simulink model "Segway3"  (R2015a)
settings: Solver=ode3  SolverMode=SingleTasking  StartTime=0.0  StopTime=10.0  RelTol=1e-3
libraries: legonxtlib x12
settings Model: ExtModeTrigDuration=2  Creator=Vladimir  LastModifiedBy=Vladimir
settings OptimizationCC: OptimizeModelRefInitCode=on  LifeSpan=1
settings DebuggingCC: UnderspecifiedInitializationDetection=Classic  MergeDetectMultiDrivingBlocksExec=none
settings HardwareCC: ProdLargestAtomicInteger=Long  ProdLargestAtomicFloat=Float  ProdEndianess=LittleEndian  ProdHWDeviceType=ARM Compatible->ARM 7
settings RTWCC: SystemTargetFile=realtime.tlc  GenerateMakefile=off  TemplateMakefile=realtime.tmf  Description=Run on Target Hardware  RTWVerbose=off
settings ERTTargetCC: CombineOutputUpdateFcns=off  ExtModeTransport=2  ExtModeMexFile=ext_serial_win32_comm_no_acks_rtt  ExtModeMexArgs=0 1 9600  ERTSrcFileBannerTemplate=realtime_code_template.cgt  ERTHdrFileBannerTemplate=realtime_code_template.cgt  ERTDataSrcFileTemplate=realtime_code_template.cgt  ERTDataHdrFileTemplate=realtime_code_template.cgt  ERTCustomFileTemplate=realtime_file_process.tlc

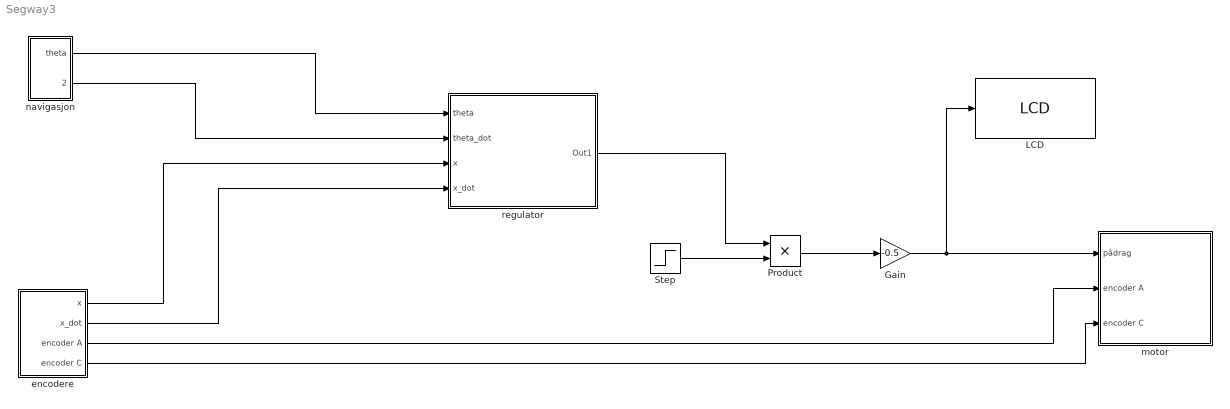
== system Segway3 ==
  Gain : Gain  Gain=-0.5
  LCD : legonxtlib/LCD  slcdStr=u  slcdLine=7  slcdFormat=Decimal  blockPlatform=LegoMindstormsNXT
  Product : Product
  Step : Step  Time=5  SampleTime=1
  encodere : Subsystem
  motor : Subsystem
  navigasjon : Subsystem
  regulator : Subsystem
  wires:
  encodere/3(encoder A) -> motor/2(encoder A)
  encodere/4("encoder C ") -> motor/3(" encoder C")
  navigasjon/1(theta) -> regulator/1(theta)
  navigasjon/2(theta_dot) -> regulator/2(theta_dot)
  encodere/1(x) -> regulator/3(x)
  encodere/2(x_dot) -> regulator/4(x_dot)
  Gain/1 -> motor/1(pådrag), LCD/1
  Step/1 -> Product/2
  regulator/1(Out1) -> Product/1
  Product/1 -> Gain/1

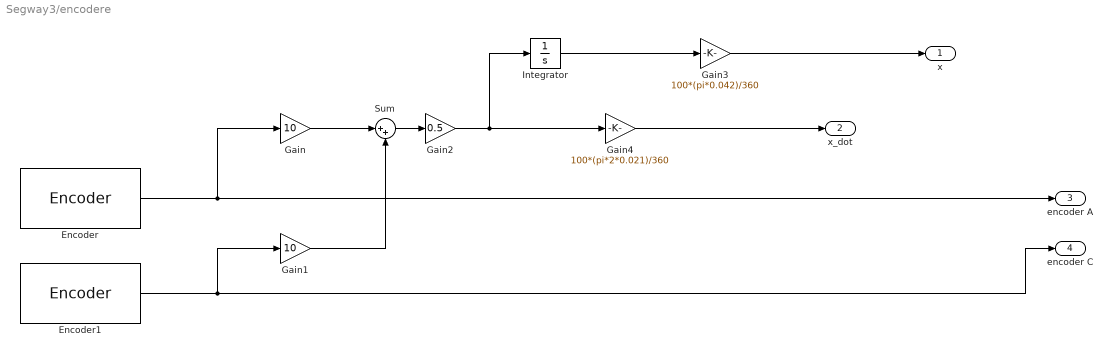
== system Segway3/encodere ==
  Encoder : legonxtlib/Encoder  portNumber=A  opMode=Reset at each sample time  sampleTime=0.1  blockPlatform=LegoMindstormsNXT
  Encoder1 : legonxtlib/Encoder  portNumber=C  opMode=Reset at each sample time  sampleTime=0.1  blockPlatform=LegoMindstormsNXT
  Gain : Gain  Gain=10
  Gain1 : Gain  Gain=10
  Gain2 : Gain  Gain=0.5  OutDataTypeStr=double
  Gain3 : Gain  Gain=100*(pi*0.042)/360
  Gain4 : Gain  Gain=100*(pi*2*0.021)/360
  Integrator : Integrator
  Sum : Sum  Inputs=|++
  x : Outport
  x_dot : Outport  Port=2
  encoder A : Outport  Port=3
  "encoder C " : Outport  Port=4
  wires:
  Encoder1/1 -> "encoder C "/1, Gain1/1
  Gain2/1 -> Gain4/1, Integrator/1
  Integrator/1 -> Gain3/1
  Sum/1 -> Gain2/1
  Gain1/1 -> Sum/2
  Gain/1 -> Sum/1
  Encoder/1 -> encoder A/1, Gain/1
  Gain3/1 -> x/1
  Gain4/1 -> x_dot/1

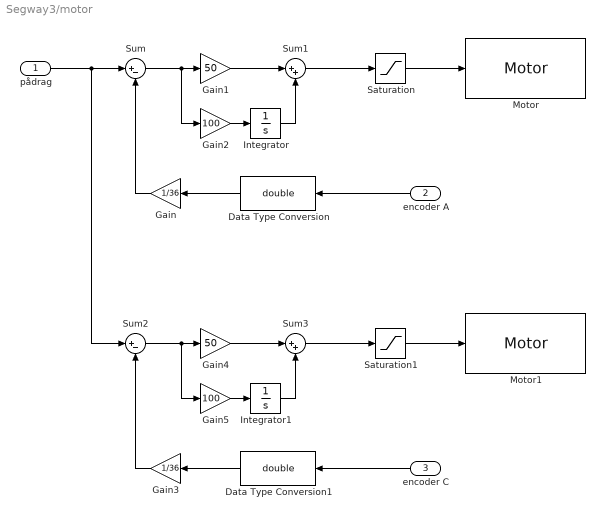
== system Segway3/motor ==
  pådrag : Inport
  encoder A : Inport  Port=2
  " encoder C" : Inport  Port=3
  Data Type Conversion : DataTypeConversion  OutDataTypeStr=double
  Data Type Conversion1 : DataTypeConversion  OutDataTypeStr=double
  Gain : Gain  Gain=1/36
  Gain1 : Gain  Gain=50
  Gain2 : Gain  Gain=100
  Gain3 : Gain  Gain=1/36
  Gain4 : Gain  Gain=50
  Gain5 : Gain  Gain=100
  Integrator : Integrator
  Integrator1 : Integrator
  Motor : legonxtlib/Motor  sportNumber=A  sstopAction=Coast  blockPlatform=LegoMindstormsNXT
  Motor1 : legonxtlib/Motor  sportNumber=C  sstopAction=Coast  blockPlatform=LegoMindstormsNXT
  Saturation : Saturate  UpperLimit=100  LowerLimit=-100
  Saturation1 : Saturate  UpperLimit=100  LowerLimit=-100
  Sum : Sum  Inputs=|+-
  Sum1 : Sum  Inputs=|++
  Sum2 : Sum  Inputs=|+-
  Sum3 : Sum  Inputs=|++
  wires:
  Saturation/1 -> Motor/1
  Data Type Conversion/1 -> Gain/1
  pådrag/1 -> Sum2/1, Sum/1
  Gain2/1 -> Integrator/1
  Integrator/1 -> Sum1/2
  Gain4/1 -> Sum3/1
  " encoder C"/1 -> Data Type Conversion1/1
  Data Type Conversion1/1 -> Gain3/1
  Sum2/1 -> Gain5/1, Gain4/1
  Gain5/1 -> Integrator1/1
  Integrator1/1 -> Sum3/2
  Sum3/1 -> Saturation1/1
  Saturation1/1 -> Motor1/1
  Gain3/1 -> Sum2/2
  Gain/1 -> Sum/2
  Sum1/1 -> Saturation/1
  Sum/1 -> Gain2/1, Gain1/1
  Gain1/1 -> Sum1/1
  encoder A/1 -> Data Type Conversion/1

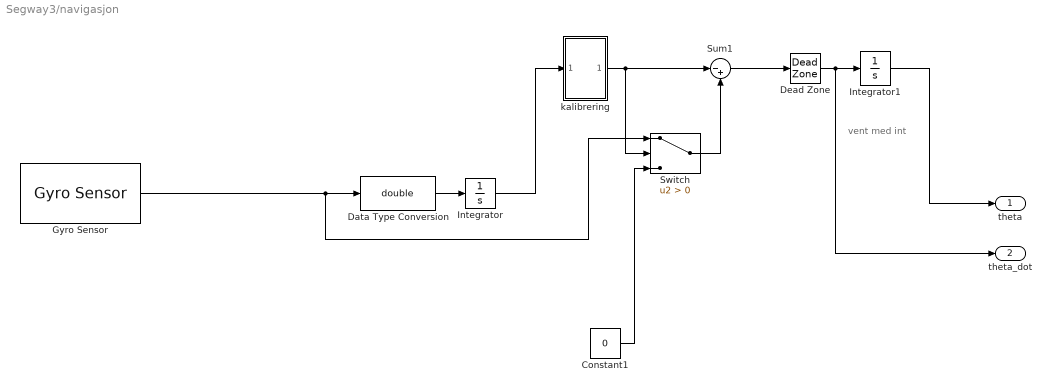
== system Segway3/navigasjon ==
  note: vent med int
  Constant1 : Constant  Value=0
  Data Type Conversion : DataTypeConversion  OutDataTypeStr=double
  Dead Zone : DeadZone  LowerValue=-1  UpperValue=1  SaturateOnIntegerOverflow=on
  Gyro Sensor : legonxtlib/Gyro Sensor  portNumber=1  outputMode=Rotation rate (-360 - 360)  offset=600  sampleTime=0.005  blockPlatform=LegoMindstormsNXT
  Integrator : Integrator
  Integrator1 : Integrator
  Sum1 : Sum  Inputs=|-+
  Switch : Switch  Criteria=u2 > Threshold
  kalibrering : Subsystem
  theta : Outport
  theta_dot : Outport  Port=2
  wires:
  Integrator1/1 -> theta/1
  Sum1/1 -> Dead Zone/1
  Data Type Conversion/1 -> Integrator/1
  Integrator/1 -> kalibrering/1(In1)
  kalibrering/1(Out1) -> Switch/2, Sum1/1
  Gyro Sensor/1 -> Switch/1, Data Type Conversion/1
  Dead Zone/1 -> theta_dot/1, Integrator1/1
  Switch/1 -> Sum1/2
  Constant1/1 -> Switch/3

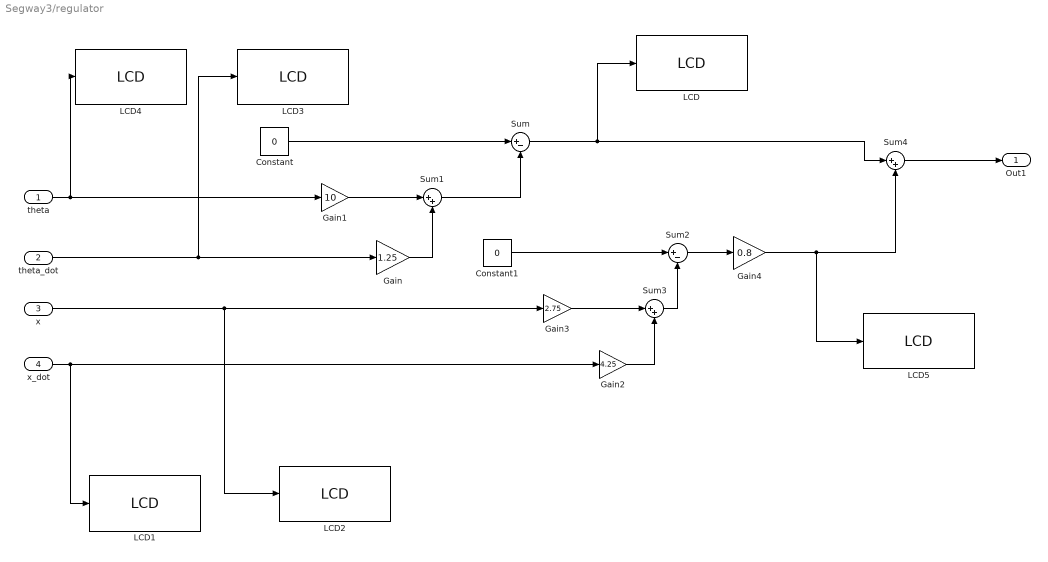
== system Segway3/regulator ==
  theta : Inport
  theta_dot : Inport  Port=2
  x : Inport  Port=3
  x_dot : Inport  Port=4
  Constant : Constant  Value=0
  Constant1 : Constant  Value=0
  Gain : Gain  Gain=1.25
  Gain1 : Gain  Gain=10
  Gain2 : Gain  Gain=4.25
  Gain3 : Gain  Gain=2.75
  Gain4 : Gain  Gain=0.8
  LCD : legonxtlib/LCD  slcdStr=gy_reg  slcdLine=5  slcdFormat=Decimal  blockPlatform=LegoMindstormsNXT
  LCD1 : legonxtlib/LCD  slcdStr=ms  slcdLine=4  slcdFormat=Decimal  blockPlatform=LegoMindstormsNXT
  LCD2 : legonxtlib/LCD  slcdStr=dis  slcdLine=3  slcdFormat=Decimal  blockPlatform=LegoMindstormsNXT
  LCD3 : legonxtlib/LCD  slcdStr=vh  slcdLine=2  slcdFormat=Decimal  blockPlatform=LegoMindstormsNXT
  LCD4 : legonxtlib/LCD  slcdStr=v  slcdLine=1  slcdFormat=Decimal  blockPlatform=LegoMindstormsNXT
  LCD5 : legonxtlib/LCD  slcdStr=en_reg  slcdLine=6  slcdFormat=Decimal  blockPlatform=LegoMindstormsNXT
  Sum : Sum  Inputs=|+-
  Sum1 : Sum  Inputs=|++
  Sum2 : Sum  Inputs=|+-
  Sum3 : Sum  Inputs=|++
  Sum4 : Sum  Inputs=|++
  Out1 : Outport
  wires:
  theta_dot/1 -> LCD3/1, Gain/1
  theta/1 -> LCD4/1, Gain1/1
  Sum4/1 -> Out1/1
  Sum1/1 -> Sum/2
  Gain/1 -> Sum1/2
  Gain2/1 -> Sum3/2
  Sum3/1 -> Sum2/2
  Constant1/1 -> Sum2/1
  Gain3/1 -> Sum3/1
  x/1 -> LCD2/1, Gain3/1
  x_dot/1 -> LCD1/1, Gain2/1
  Constant/1 -> Sum/1
  Sum/1 -> LCD/1, Sum4/1
  Gain1/1 -> Sum1/1
  Sum2/1 -> Gain4/1
  Gain4/1 -> LCD5/1, Sum4/2

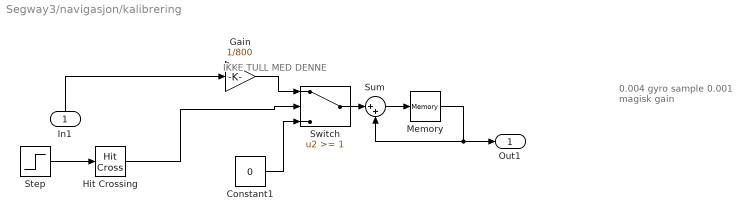
== system Segway3/navigasjon/kalibrering ==
  note: 0.004 gyro sample
      | 0.001 magisk gain
  note: IKKE TULL MED DENNE
  In1 : Inport
  Constant1 : Constant  Value=0
  Gain : Gain  Gain=1/800
  Hit Crossing : HitCross  HitCrossingOffset=0.5
  Memory : Memory
  Step : Step  Time=4  SampleTime=1
  Sum : Sum  Inputs=|++
  Switch : Switch  Threshold=1
  Out1 : Outport
  wires:
  Memory/1 -> Out1/1, Sum/2
  Gain/1 -> Switch/1
  Step/1 -> Hit Crossing/1
  Constant1/1 -> Switch/3
  Sum/1 -> Memory/1
  Hit Crossing/1 -> Switch/2
  Switch/1 -> Sum/1
  In1/1 -> Gain/1
